simulink model "LIPO"  (R2022b)
settings: Solver=ode1  StartTime=0.0  StopTime=3000  FixedStep=1e-3  RelTol=1e-3
values from neighbouring files (symbols this model uses):
  c_bat = 9.3    [init_bat.m]
  cl = [1483.05084746 5264.83050847 7934.3220339 9841.10169492 10858.0508475 11875 12701.2711864 13146.1864407 13591.1016949 13908.8983051 14163.1355932 14385.5932203 ... (42 elements, 42x1)]    [cl.mat]
  cs = [1603.2888 2639.26 3588.9004 4522.0967 4982.5283 5303.186 5459.404 5607.4 5730.7295 5829.3936 5895.1694 5936.28 ... (38 elements, 38x1)]    [cs.mat]
  eff = 0.99    [init_bat.m]
  ri = [0.010884774 0.009979424 0.009341564 0.008765432 0.008333334 0.008065844 0.007880659 0.007757202 0.007654321 0.0076131686 0.0076131686 0.0075720167 ... (26 elements, 26x1)]    [ri.mat]
  rl = [0.03391949 0.027415255 0.020338982 0.013220339 0.009152543 0.0077966102 0.0065762713 0.005940678 0.0054067797 0.0050508473 0.004745763 0.0045423727 ... (39 elements, 39x1)]    [rl.mat]
  rs = [0.004855263 0.004289474 0.0034605262 0.0028289473 0.0022105263 0.0018947369 0.0016578947 0.0014473684 0.0012763158 0.0011315789 0.0010131579 0.00092105265 ... (33 elements, 33x1)]    [rs.mat]
  soc_0 = 100    [init_bat.m]
  soc_cl = [-0.192307692308 2.88461538462 5.0641025641 6.66666666667 7.69230769231 8.91025641026 10.1923076923 11.4743589744 13.7179487179 17.0512820513 19.8076923077 22.2435897436 ... (42 elements, 42x1)]    [soc_cl.mat]
  soc_cs = [-0.7744875 3.4624145 7.5626426 11.731207 14.191344 16.036446 17.334852 18.838268 20.341686 22.209568 24.53303 26.90205 ... (38 elements, 38x1)]    [soc_cs.mat]
  soc_ri = [-0.07874016 3.03937 5.3070865 7.6692915 9.748032 11.92126 14.755905 17.496063 21.559055 25.338583 29.874016 35.44882 ... (26 elements, 26x1)]    [soc_ri.mat]
  soc_rl = [-1.2052118 1.1617807 3.6373508 6.330076 7.937025 8.5884905 9.309446 9.908794 10.560261 11.1074915 12.28013 14.521173 ... (39 elements, 39x1)]    [soc_rl.mat]
  soc_rs = [0 1.3372093 3.4302325 5 6.918605 7.9651165 8.924418 9.709302 10.843023 12.063953 13.633721 15.726745 ... (33 elements, 33x1)]    [soc_rs.mat]
  soc_voc = [-1.1339012 2.7481961 4.883472 5.5628567 6.436503 7.374857 8.280936 8.992884 9.899058 11.323137 13.362287 15.239641 ... (40 elements, 40x1)]    [soc_voc.mat]
  voc = [2.896806 3.0302253 3.0969358 3.1193313 3.1398218 3.1622183 3.1793738 3.1912878 3.2032024 3.217025 3.229897 3.2394333 ... (40 elements, 40x1)]    [voc.mat]
settings Model: Creator=habayah  LastModifiedBy=ZinouAb
settings ModelReferenceCC: EnableRefExpFcnMdlSchedulingChecks=on

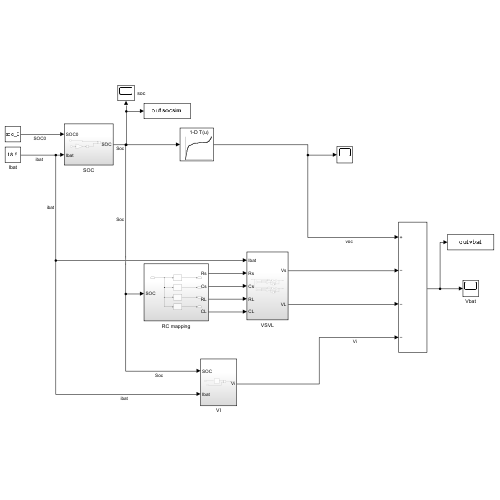
[thumbnail: Simulink's stored preview of the top-level diagram]
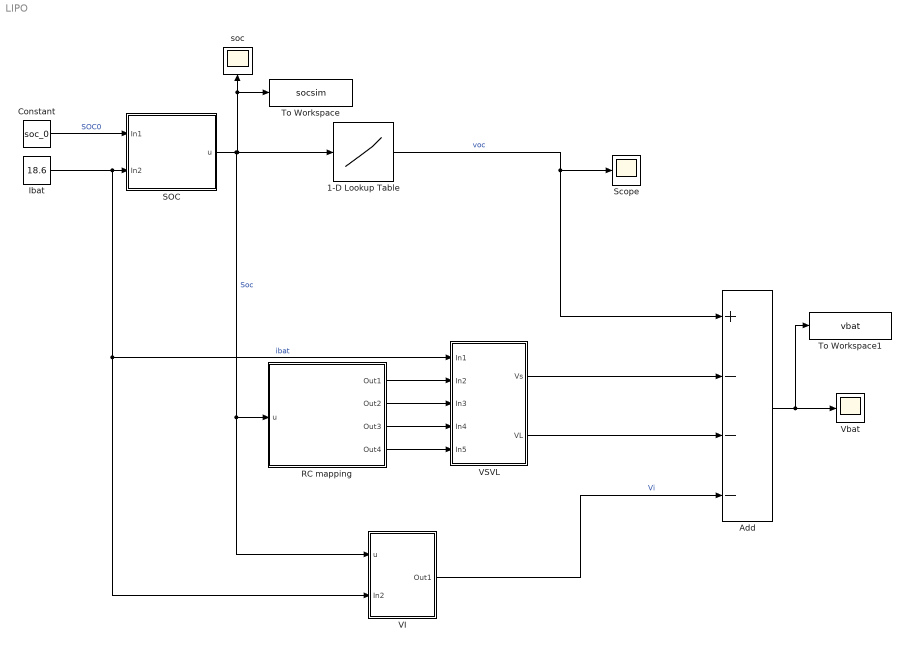
== system LIPO ==
  1-D Lookup Table : Lookup_n-D  NumberOfTableDimensions=1  BreakpointsForDimension1=soc_voc  Table=voc  InternalRulePriority=Speed  RndMeth=Simplest
  Add : Sum  Inputs=+---
  Constant : Constant  Value=soc_0
  Ibat : Constant  Value=18.6
  RC mapping : Subsystem
  SOC : Subsystem
  Scope : Scope
  To Workspace : ToWorkspace  VariableName=socsim  SaveFormat=Timeseries  SampleTime=-1
  To Workspace1 : ToWorkspace  VariableName=vbat  SaveFormat=Timeseries  SampleTime=-1
  VI : Subsystem
  VSVL : Subsystem
  Vbat : Scope
  soc : Scope
  wires:
  SOC/1(u) -> 1-D Lookup Table/1, To Workspace/1, soc/1, VI/1(u), RC mapping/1(u)  "Soc"
  Constant/1 -> SOC/1(In1)  "SOC0"
  Ibat/1 -> VI/2(In2), VSVL/1(In1), SOC/2(In2)  "ibat"
  RC mapping/1(Out1) -> VSVL/2(In2)
  RC mapping/2(Out2) -> VSVL/3(In3)
  RC mapping/3(Out3) -> VSVL/4(In4)
  RC mapping/4(Out4) -> VSVL/5(In5)
  VI/1(Out1) -> Add/4  "Vi"
  1-D Lookup Table/1 -> Add/1, Scope/1  "voc"
  VSVL/1(Vs) -> Add/2
  VSVL/2(VL) -> Add/3
  Add/1 -> To Workspace1/1, Vbat/1

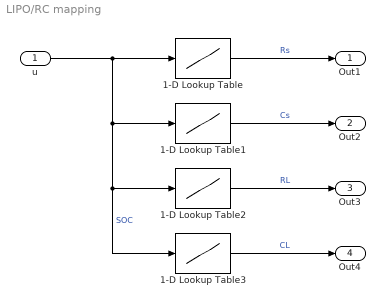
== system LIPO/RC mapping ==
  u : Inport
  1-D Lookup Table : Lookup_n-D  NumberOfTableDimensions=1  BreakpointsForDimension1=soc_rs  Table=rs  InternalRulePriority=Speed  RndMeth=Simplest
  1-D Lookup Table1 : Lookup_n-D  NumberOfTableDimensions=1  BreakpointsForDimension1=soc_cs  Table=cs  InternalRulePriority=Speed  RndMeth=Simplest
  1-D Lookup Table2 : Lookup_n-D  NumberOfTableDimensions=1  BreakpointsForDimension1=soc_rl  Table=rl  InternalRulePriority=Speed  RndMeth=Simplest
  1-D Lookup Table3 : Lookup_n-D  NumberOfTableDimensions=1  BreakpointsForDimension1=soc_cl  Table=cl  InternalRulePriority=Speed  RndMeth=Simplest
  Out1 : Outport
  Out2 : Outport  Port=2
  Out3 : Outport  Port=3
  Out4 : Outport  Port=4
  wires:
  1-D Lookup Table2/1 -> Out3/1  "RL"
  1-D Lookup Table1/1 -> Out2/1  "Cs"
  u/1 -> 1-D Lookup Table3/1, 1-D Lookup Table2/1, 1-D Lookup Table1/1, 1-D Lookup Table/1  "SOC"
  1-D Lookup Table/1 -> Out1/1  "Rs"
  1-D Lookup Table3/1 -> Out4/1  "CL"

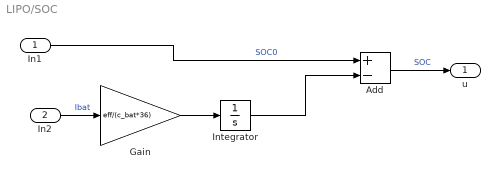
== system LIPO/SOC ==
  In1 : Inport
  In2 : Inport  Port=2
  Add : Sum  Inputs=+-
  Gain : Gain  Gain=eff/(c_bat*36)
  Integrator : Integrator
  u : Outport
  wires:
  Integrator/1 -> Add/2
  In1/1 -> Add/1  "SOC0"
  Gain/1 -> Integrator/1
  Add/1 -> u/1  "SOC"
  In2/1 -> Gain/1  "Ibat"

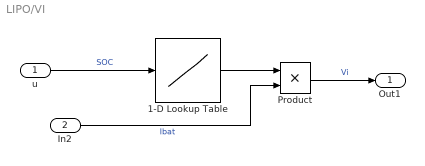
== system LIPO/VI ==
  u : Inport
  In2 : Inport  Port=2
  1-D Lookup Table : Lookup_n-D  NumberOfTableDimensions=1  BreakpointsForDimension1=soc_ri  Table=ri  InternalRulePriority=Speed  RndMeth=Simplest
  Product : Product
  Out1 : Outport
  wires:
  u/1 -> 1-D Lookup Table/1  "SOC"
  1-D Lookup Table/1 -> Product/1
  In2/1 -> Product/2  "Ibat"
  Product/1 -> Out1/1  "Vi"

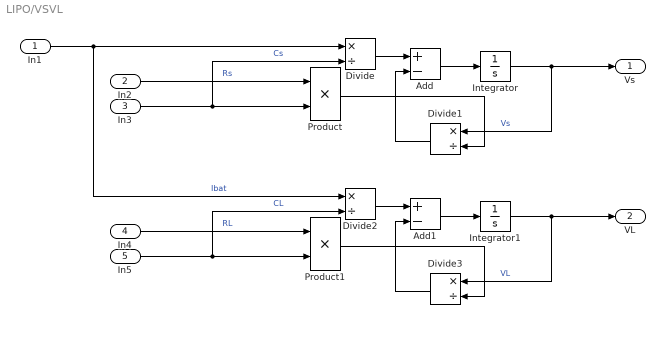
== system LIPO/VSVL ==
  In1 : Inport
  In2 : Inport  Port=2
  In3 : Inport  Port=3
  In4 : Inport  Port=4
  In5 : Inport  Port=5
  Add : Sum  Inputs=+-
  Add1 : Sum  Inputs=+-
  Divide{,1..3} (4 alike) : Product  Inputs=*/
  Integrator : Integrator
  Integrator1 : Integrator
  Product : Product
  Product1 : Product
  Vs : Outport
  VL : Outport  Port=2
  wires:
  Product/1 -> Divide1/2
  Integrator/1 -> Vs/1, Divide1/1  "Vs"
  Divide1/1 -> Add/2
  Divide/1 -> Add/1
  Add/1 -> Integrator/1
  In3/1 -> Divide/2, Product/2  "Cs"
  In2/1 -> Product/1  "Rs"
  In5/1 -> Divide2/2, Product1/2  "CL"
  In4/1 -> Product1/1  "RL"
  In1/1 -> Divide2/1, Divide/1  "Ibat"
  Divide2/1 -> Add1/1
  Add1/1 -> Integrator1/1
  Divide3/1 -> Add1/2
  Integrator1/1 -> VL/1, Divide3/1  "VL"
  Product1/1 -> Divide3/2
